simulink model "Lab2"  (R2022b)
settings: Solver=FixedStepAuto  StartTime=0.0  StopTime=10.0  RelTol=1e-3
values from neighbouring files (symbols this model uses):
  g = 9.81    [InitModel.m]
  l = 5    [InitModel.m]
  theta0 = 0    [InitModel.m]
  theta_dot0 = pi/4    (= 0.785398163397)    [InitModel.m]
settings Model: Creator=filippocamaleonte  LastModifiedBy=filippocamaleonte

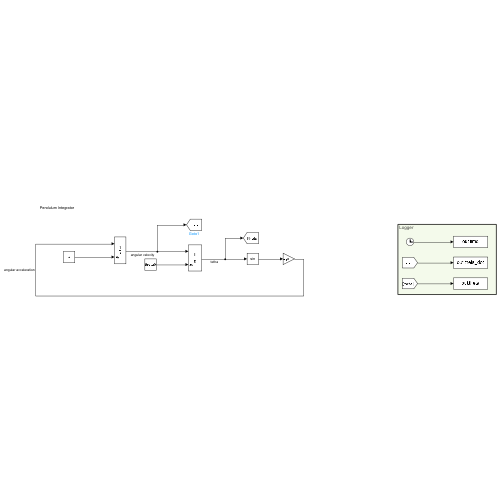
[thumbnail: Simulink's stored preview of the top-level diagram]
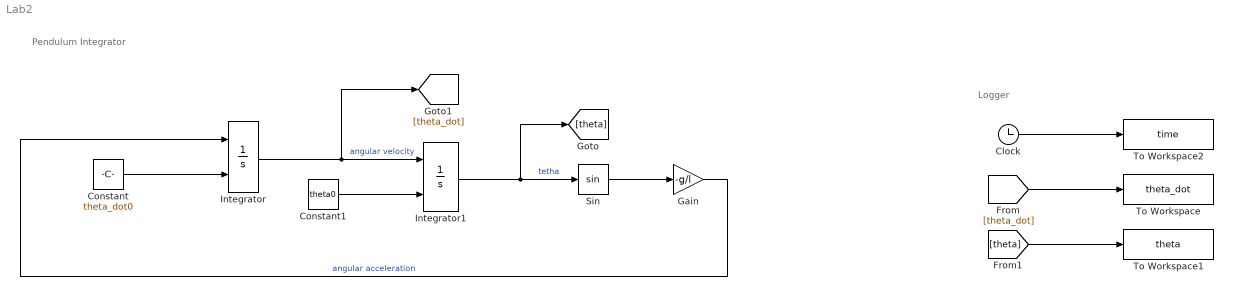
== system Lab2 ==
  note: Logger
  note: Pendulum Integrator
  Clock : Clock
  Constant : Constant  Value=theta_dot0
  Constant1 : Constant  Value=theta0
  Gain : Gain  Gain=-g/l
  Integrator : Integrator  InitialConditionSource=external
  Integrator1 : Integrator  InitialConditionSource=external
  Sin : Trigonometry
  To Workspace : ToWorkspace  VariableName=theta_dot  SaveFormat=Timeseries  SampleTime=-1
  To Workspace1 : ToWorkspace  VariableName=theta  SaveFormat=Timeseries  SampleTime=-1
  To Workspace2 : ToWorkspace  VariableName=time  SaveFormat=Timeseries  SampleTime=-1
  wires:
  Integrator/1 -> [theta_dot], Integrator1/1  "angular velocity"
  Gain/1 -> Integrator/1  "angular acceleration"
  Integrator1/1 -> [theta], Sin/1  "tetha"
  Constant/1 -> Integrator/2
  Constant1/1 -> Integrator1/2
  Sin/1 -> Gain/1
  Clock/1 -> To Workspace2/1
  [theta_dot] -> To Workspace/1
  [theta] -> To Workspace1/1
